simulink model "ERMAX228"  (R2019b)
settings: Solver=VariableStepAuto  StartTime=0.0  StopTime=10.0  RelTol=1e-3
model workspace (MAT data in the model file):
  Eff = [83  84  85  84.5  85  84.8  84.6  84.3  84  83.5  82.8; 84  84  86  86  85.8  85.6  85.6  85.2  84.5  84  83.3; 84  86  87.5  88  88  88  87  86  85  84.5  83.9; 84  87  88.5  90  91  91  90  88  86.2  85.5  84.5; 84  87.5  89.5  93.8  93.5  93.8  94.3  91  89.5  86.5  85; 84  88  92  94.2  94.5  94.5  95  94  91  91.5  85.8; 84  88  92.5  94.6  95  95.3  95.4  94.7  92  90.2  85.8; 84  88  93  95.6  96.2  96.3  95.4  94.9  93  90.2  85.5; 84  88  93  95.8  96.4  97  95.4  94.9  94  90.2  85.8; 84  88  92  96  96.6  97.5  95.4  94.9  94  90.2  85.8; 84  88  93  95.9  98  97.5  95.4  94.9  94  90.2  85.8; 84  88  93  95.9  97.5  97.5  95.4  94.9  94  90.2  85.8; 84  88  93  95.6  97  97.5  95.4  94.9  94  90.2  85.8; 84  88  93  95.5  96.8  97.3  95.4  94.9  94  90.2  85.8; 84  86  93  95  96.4  96.5  95.4  94.9  94  90.2  85.8; 83.5  85  93  94.8  96.2  96.2  95.4  94.8  94  90.2  85.8; 83.5  84  92  94.6  95.7  95.7  95.2  94.8  94  90.2  85.8; 83.2  83.5  89.5  94.4  95.2  95.5  95.1  94.7  94  90.2  85.8; 83  83.2  88  94  94.7  95.2  95  94.6  94  90.2  85.8; 82.7  83  86  91  94.3  94.5  94.8  94.6  94  90.2  85.8; 82.5  83.7  85  92  93.8  94.2  94.5  94.5  94  90.2  85.8; 82.3  83.4  84  90  90  93  94.3  94.3  94  90.2  85.8; 82  82.7  83  84  85.2  86  94  94  94  90.2  85.8]
  MtrSpd_sample = [0 1200 1400 1600 1800 2000 2200 2400 2600 2800 3000 3200 3400 3600 3800 4000 4200 4400 4600 4800 5000 6000 7000]
  MtrTrq_sample = [240 240 240 240 240 240 240 239.1 237.8 236.6 235.7 234.5 233.1 231.6 230.6 228 225.8 222.9 220.6 217.7 216.2 216 216]
  Spd = [0 250 500 750 1000 1250 1500 1750 2000 2250 2500 2750 3000 3250 3500 3750 4000 4250 4500 4750 5000 5250 5500]
  Tc = 0.02
  Trq = [0 25 50 75 100 125 150 175 200 225 250]
settings Model: OrderedModelArguments=off  Creator=ZHOU Jinhan  LastModifiedBy=ZHOU Jinhan

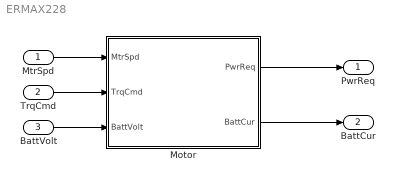
== system ERMAX228 ==
  MtrSpd : Inport
  TrqCmd : Inport  Port=2
  BattVolt : Inport  Port=3
  Motor : Subsystem  mask{Eff=[83 84 85 84.5 85 84.8 84.59999999999999 84.3 84 83.5 82.8;84 84 86 86 85.8 85.59999999999999 85.59999999999999 85.2 84.5 84 83.3;84 86 87.5 88 88 88 87 86 85 84.5 83.90000000000001;84 87 88.5 90 91 91 90 88 86.2 85.5 84.5;84 87.5 89.5 93.8 93.5 93.8 94.3 91 89.5 86.5 85;84 88 92 94.2 94.5 94.5 95 94 91 91.5 85.8;84 88 92.5 94.59999999999999 95 95.3 95.40000000000001 94.7 92 90.2 85.8;84 88 93 95.59999999999999 96.2 96.3 95.40000000000001 94.90000000000001 93 90.2 85.5;84 88 93 95.8 96.40000000000001 97 95.40000000000001 94.90000000000001 94 90.2 85.8;84 88 92 96 96.59999999999999 97.5 95.40000000000001 94.90000000000001 94 90.2 85.8;84 88 93 95.90000000000001 98 97.5 95.40000000000001 94.90000000000001 94 90.2 85.8;84 88 93 95.90000000000001 97.5 97.5 95.40000000000001 94.90000000000001 94 90.2 85.8;84 88 93 95.59999999999999 97 97.5 95.40000000000001 94.90000000000001 94 90.2 85.8;84 88 93 95.5 96.8 97.3 95.40000000000001 94.90000000000001 94 90.2 85.8;84 86 93 95 96.40000000000001 96.5 95.40000000000001 94.90000000000001 94 90.2 85.8;83.5 85 93 94.8 96.2 96.2 95.40000000000001 94.8 94 90.2 85.8;83.5 84 92 94.59999999999999 95.7 95.7 95.2 94.8 94 90.2 85.8;83.2 83.5 89.5 94.40000000000001 95.2 95.5 95.09999999999999 94.7 94 90.2 85.8;83 83.2 88 94 94.7 95.2 95 94.59999999999999 94 90.2 85.8;82.7 83 86 91 94.3 94.5 94.8 94.59999999999999 94 90.2 85.8;82.5 83.7 85 92 93.8 94.2 94.5 94.5 94 90.2 85.8;82.3 83.40000000000001 84 90 90 93 94.3 94.3 94 90.2 85.8;82 82.7 83 84 85.2 86 94 94 94 90.2 85.8], MtrSpd_sample=[0 1200 1400 1600 1800 2000 2200 2400 2600 2800 3000 3200 3400 3600 3800 4000 4200 4400 4600 4800 5000 6000 7000], MtrTrq_sample=[240 240 240 240 240 240 240 239.1 237.8 236.6 235.7 234.5 233.1 231.6 230.6 228 225.8 222.9 220.6 217.7 216.2 216 216], Spd=[0 250 500 750 1000 1250 1500 1750 2000 2250 2500 2750 3000 3250 3500 3750 4000 4250 4500 4750 5000 5250 5500], Tc=0.02, Trq=[0 25 50 75 100 125 150 175 200 225 250]}
      mask Display: image('$imagefile'); % Use "Edit Image" on toolstrip to change.
  PwrReq : Outport
  BattCur : Outport  Port=2
  wires:
  MtrSpd/1 -> Motor/1(MtrSpd)
  Motor/1(PwrReq) -> PwrReq/1
  Motor/2(BattCur) -> BattCur/1
  TrqCmd/1 -> Motor/2(TrqCmd)
  BattVolt/1 -> Motor/3(BattVolt)

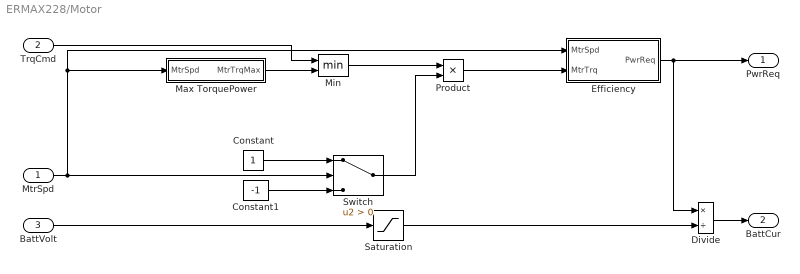
== system ERMAX228/Motor ==
  MtrSpd : Inport
  TrqCmd : Inport  Port=2
  BattVolt : Inport  Port=3
  Constant : Constant
  Constant1 : Constant  Value=-1
  Divide : Product  Inputs=*/
  Efficiency : Subsystem
  Max TorquePower : Subsystem
  Min : MinMax  Inputs=2
  Product : Product
  Saturation : Saturate  UpperLimit=Inf  LowerLimit=0.001
  Switch : Switch  Criteria=u2 > Threshold
  PwrReq : Outport
  BattCur : Outport  Port=2
  wires:
  MtrSpd/1 -> Efficiency/1(MtrSpd), Max TorquePower/1(MtrSpd), Switch/2
  Efficiency/1(PwrReq) -> Divide/1, PwrReq/1
  Constant1/1 -> Switch/3
  Constant/1 -> Switch/1
  Min/1 -> Product/1
  Product/1 -> Efficiency/2(MtrTrq)
  Max TorquePower/1(MtrTrqMax) -> Min/2
  TrqCmd/1 -> Min/1
  Switch/1 -> Product/2
  Divide/1 -> BattCur/1
  BattVolt/1 -> Saturation/1
  Saturation/1 -> Divide/2

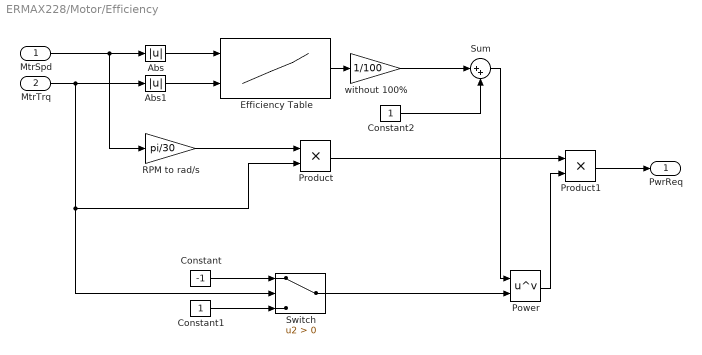
== system ERMAX228/Motor/Efficiency ==
  MtrSpd : Inport
  MtrTrq : Inport  Port=2
  Abs : Abs
  Abs1 : Abs
  Constant : Constant  Value=-1
  Constant1 : Constant
  Constant2 : Constant
  Efficiency Table : Lookup_n-D  LookupTableObject=Efficiency  BreakpointsForDimension1=Spd  BreakpointsForDimension2=Trq  Table=Eff  InterpMethod=Linear Lagrange  InternalRulePriority=Speed  RndMeth=Simplest  InputSameDT=on
  Power : Math  Operator=pow  SignedPower=off  SaturateOnIntegerOverflow=on
  Product : Product
  Product1 : Product
  RPM to rad/s : Gain  Gain=pi/30
  Sum : Sum  Inputs=|++
  Switch : Switch  Criteria=u2 > Threshold
  without 100% : Gain  Gain=1/100
  PwrReq : Outport
  wires:
  MtrSpd/1 -> RPM to rad/s/1, Abs/1
  MtrTrq/1 -> Switch/2, Product/2, Abs1/1
  Efficiency Table/1 -> without 100%/1
  Sum/1 -> Power/1
  Abs/1 -> Efficiency Table/1
  Abs1/1 -> Efficiency Table/2
  without 100%/1 -> Sum/1
  Constant/1 -> Switch/1
  Constant1/1 -> Switch/3
  Switch/1 -> Power/2
  RPM to rad/s/1 -> Product/1
  Constant2/1 -> Sum/2
  Product/1 -> Product1/1
  Power/1 -> Product1/2
  Product1/1 -> PwrReq/1

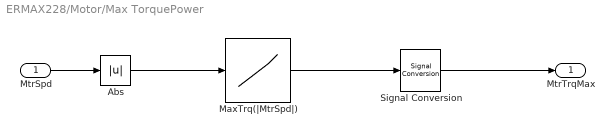
== system ERMAX228/Motor/Max TorquePower ==
  MtrSpd : Inport
  Abs : Abs
  MaxTrq(|MtrSpd|) : Lookup_n-D  NumberOfTableDimensions=1  BreakpointsForDimension1=MtrSpd_sample  Table=MtrTrq_sample  InterpMethod=Linear Lagrange  InternalRulePriority=Speed  RndMeth=Simplest  InputSameDT=on
  Signal Conversion : SignalConversion  OverrideOpt=off
  MtrTrqMax : Outport
  wires:
  Abs/1 -> MaxTrq(|MtrSpd|)/1
  MaxTrq(|MtrSpd|)/1 -> Signal Conversion/1
  Signal Conversion/1 -> MtrTrqMax/1
  MtrSpd/1 -> Abs/1
